simulink model "dyn_alloc_demo"  (Simulink 5.1)
settings: Solver=ode45  StartTime=0.0  StopTime=10.0  RelTol=1e-3
libraries: qcatlib x1
settings Model: Creator=ola  LastModifiedBy=ola  ExtModeAutoUpdateStatusClock=off  ProdHWDeviceType=Microprocessor

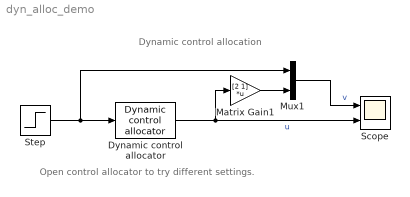
== system dyn_alloc_demo ==
  note: Dynamic control allocation
  note: Open control allocator to try different settings.
  Dynamic control allocator : qcatlib/Dynamic control allocator  B=[2 1]  plim=[-1 1;-1 1]  rlim=[-1 1;-5 5]  T=.1  Wv=1  W1=diag([1 1])  W2=diag([8 0])  S=[.5 0]'
  Matrix Gain1 : Gain  Gain=[2 1]  Multiplication=Matrix(K*u)  SaturateOnIntegerOverflow=on
  Mux1 : Mux  Inputs=2
  Scope : Scope  NumInputPorts=2
      settings: TimeRange=10  YMin=0~0  YMax=1.2~1
  Step : Step  SampleTime=0
  wires:
  Matrix Gain1/1 -> Mux1/2
  Dynamic control allocator/1 -> Matrix Gain1/1, Scope/2  "u"
  Mux1/1 -> Scope/1  "v"
  Step/1 -> Mux1/1, Dynamic control allocator/1
